simulink model "LineSensor"  (R2018b)
settings: Solver=FixedStepDiscrete  StartTime=0.0  StopTime=inf  RelTol=1e-3
model workspace (MAT data in the model file):
  InsideGain = Simulink.Parameter
  InsideGain.Value = 4
  InsideGain.DataType = 'auto'
  InsideGain.Dimensions = [1 1]
  OutsideGain = Simulink.Parameter
  OutsideGain.Value = 7
  OutsideGain.DataType = 'auto'
  OutsideGain.Dimensions = [1 1]
settings Model: Creator=Apocalypse  LastModifiedBy=Apocalypse
settings OptimizationCC: DefaultParameterBehavior=Inlined  UseDivisionForNetSlopeComputation=on  UseFloatMulNetSlope=on  PassReuseOutputArgsAs=Individual arguments  ZeroExternalMemoryAtStartup=off  ZeroInternalMemoryAtStartup=off  NoFixptDivByZeroProtection=on  EfficientFloat2IntCast=on  LifeSpan=1  OptimizeBlockOrder=speed  DifferentSizesBufferReuse=on
settings DebuggingCC: ParameterTunabilityLossMsg=error
settings HardwareCC: ProdBitPerInt=16  ProdBitPerPointer=16  ProdBitPerSizeT=16  ProdBitPerPtrDiffT=16  ProdLargestAtomicFloat=None  ProdWordSize=8  ProdLongLongMode=on  ProdHWDeviceType=Atmel->AVR
settings SFSimCC: MATLABDynamicMemAlloc=off
settings RTWCC: SystemTargetFile=ert.tlc  GenCodeOnly=on  TemplateMakefile=ert_default_tmf  GenerateReport=on  BuildConfiguration=Faster Runs  IncludeHyperlinkInReport=on  LaunchReport=on  GenerateTraceInfo=on  GenerateTraceReport=on  GenerateTraceReportSl=on  GenerateTraceReportSf=on  GenerateTraceReportEml=on
settings RTWCC: CustomSourceCode=|
  | int LeftLuminanceOutsideData[5];
  | int LeftLuminanceInsideData[5];
  | int RightLuminanceInsideData[5];
  | int RightLuminanceOutsideData[5];
  | 
  | void GetLuminance(void)
  | {
  |     LeftLuminanceInside = analogRead(LEFT_LINE_PATROL_INSIDE_SENSOR);
  |     RightLuminanceInside = analogRead(RIGHT_LINE_PATROL_INSIDE_SENSOR);
  |     LeftLuminanceOutside = analogRead(LEFT_LINE_PATROL_OUTSIDE_SENSOR);
  |     RightLuminanceOutside = analogRead(RIGHT_LINE_PATROL_OUTSIDE_SENSOR);
  | }
settings RTWCC: CustomHeaderCode=|
  | #include <SPI.h>
  | extern const int LEFT_LINE_PATROL_OUTSIDE_SENSOR;
  | extern const int LEFT_LINE_PATROL_INSIDE_SENSOR;
  | extern const int RIGHT_LINE_PATROL_INSIDE_SENSOR;
  | extern const int RIGHT_LINE_PATROL_OUTSIDE_SENSOR;
  | extern void GetLuminance(void);
settings RTWCC: CustomInitializer=|
  | pinMode(LEFT_LINE_PATROL_OUTSIDE_SENSOR, INPUT);
  | pinMode(LEFT_LINE_PATROL_INSIDE_SENSOR, INPUT);
  | pinMode(RIGHT_LINE_PATROL_INSIDE_SENSOR, INPUT);
  | pinMode(RIGHT_LINE_PATROL_OUTSIDE_SENSOR, INPUT);
settings CodeAppCC: GenerateComments=off  IgnoreCustomStorageClasses=off  OperatorAnnotations=on  SimulinkDataObjDesc=on  SFDataObjDesc=on  CustomSymbolStrGlobalVar=rt$R$N$M  CustomSymbolStrType=$R$N$M  CustomSymbolStrFcn=$N$M$F  CustomSymbolStrMacro=$N$M  InsertBlockDesc=on
settings ERTTargetCC: TargetLangStandard=C99 (ISO)  CombineSignalStateStructs=on  SuppressErrorStatus=on  SupportAbsoluteTime=off  SupportComplex=off  InlinedParameterPlacement=NonHierarchical  RootIOFormat=Structure reference  ERTCustomFileTemplate=example_file_process.tlc  ERTFilePackagingFormat=Compact

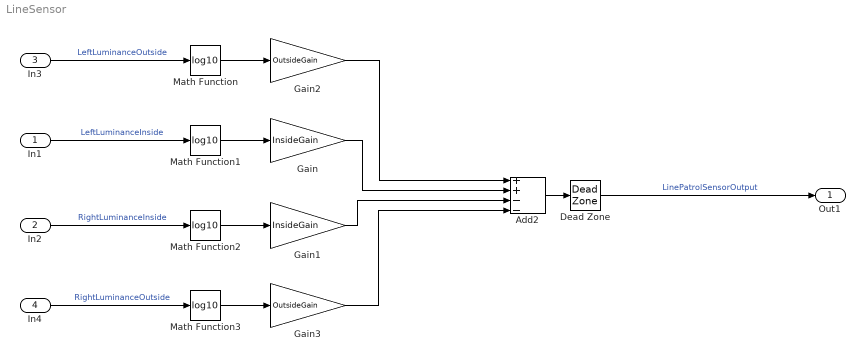
== system LineSensor ==
  In1 : Inport
  In2 : Inport  Port=2
  In3 : Inport  Port=3
  In4 : Inport  Port=4
  Add2 : Sum  Inputs=++--
  Dead Zone : DeadZone  LowerValue=-0.4  UpperValue=0.4  SaturateOnIntegerOverflow=on
  Gain : Gain  Gain=InsideGain
  Gain1 : Gain  Gain=InsideGain
  Gain2 : Gain  Gain=OutsideGain
  Gain3 : Gain  Gain=OutsideGain
  Math Function{,1..3} (4 alike) : Math  Operator=log10  SaturateOnIntegerOverflow=on
  Out1 : Outport
  wires:
  In1/1 -> Math Function1/1  "LeftLuminanceInside"
  In2/1 -> Math Function2/1  "RightLuminanceInside"
  Gain/1 -> Add2/2
  Gain1/1 -> Add2/3
  In3/1 -> Math Function/1  "LeftLuminanceOutside"
  Gain2/1 -> Add2/1
  In4/1 -> Math Function3/1  "RightLuminanceOutside"
  Gain3/1 -> Add2/4
  Dead Zone/1 -> Out1/1  "LinePatrolSensorOutput"
  Math Function/1 -> Gain2/1
  Math Function1/1 -> Gain/1
  Math Function2/1 -> Gain1/1
  Math Function3/1 -> Gain3/1
  Add2/1 -> Dead Zone/1
